simulink model "quadr_function"  (R2025b)
settings: Solver=VariableStepAuto  StartTime=0.0  StopTime=20  RelTol=1e-3
undefined symbols (not defined in the file or in its folder): K_att
libraries: mpclib x1
settings Model: Creator=abhay  LastModifiedBy=abhay

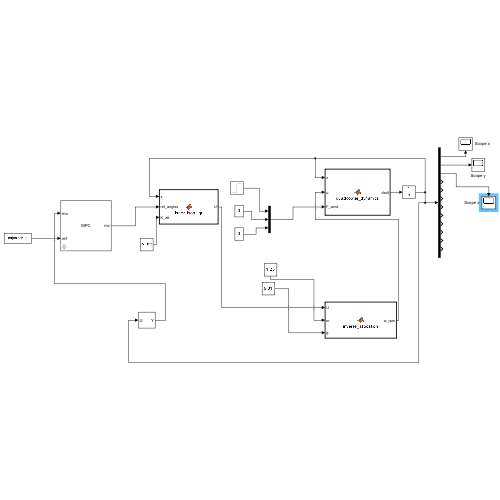
[thumbnail: Simulink's stored preview of the top-level diagram]
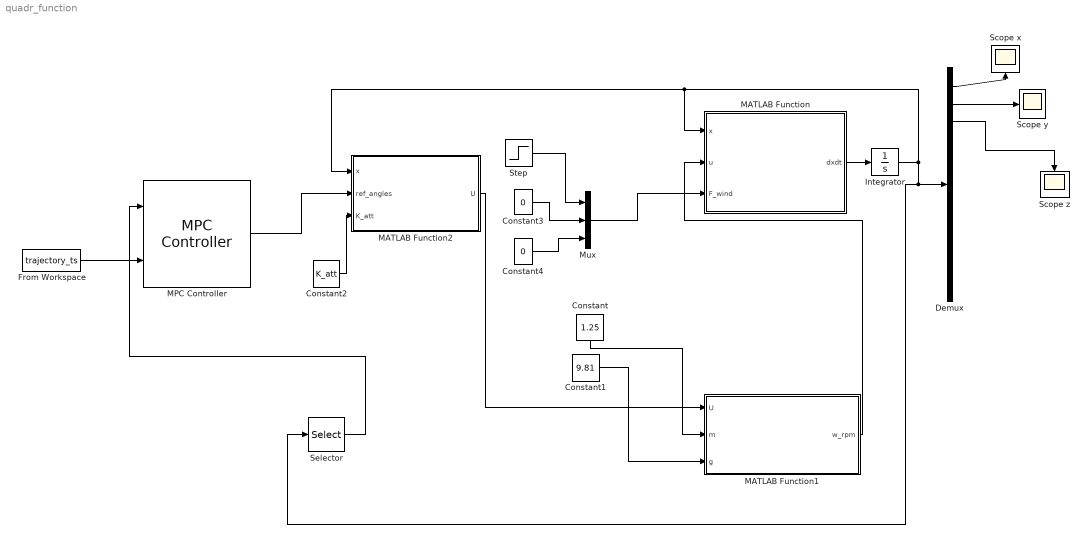
== system quadr_function ==
  Constant : Constant  Value=1.25
  Constant1 : Constant  Value=9.81
  Constant2 : Constant  Value=K_att  VectorParams1D=off
  Constant3 : Constant  Value=0
  Constant4 : Constant  Value=0
  Demux : Demux  Outputs=12
  From Workspace : FromWorkspace  VariableName=trajectory_ts
  Integrator : Integrator  InitialCondition=[2; 0; 10; 0; 1.0; 0.5; 0; 0; 0; 0; 0; 0]
  MATLAB Function : MATLAB Function  TreatAsAtomicUnit=on
  MATLAB Function1 : MATLAB Function  TreatAsAtomicUnit=on
  MATLAB Function2 : MATLAB Function  TreatAsAtomicUnit=on
  MPC Controller : mpclib/MPC Controller  SCDEnableBlockLinearizationSpecification=on  mpcobj=mpcobj  is_multiple=0  enable_value=0  return_u0=off  updateMPCinCallerWorkspace=on  md_inport=off  mv_inport=off  uref_inport=off  return_cost=off  return_mvseq=off  return_qpstatus=off  return_xseq=off  return_state=off  return_ovseq=off  state_inport=off  umin_inport=off  umax_inport=off  ymin_inport=off  ymax_inport=off  cc_inport=off  ywt_inport=off  uwt_inport=off  duwt_inport=off  rhoeps_inport=off  pm_inport=off  MaximumP=10  HorizonChoice=FixedHorizon  n_ts=0.05  n_p=20  n_mv=3  n_md=0  n_ud=0  n_mo=6  n_uo=0  BlockDataType=double  SampleTimeInherited=off  switch_inport=off
  Mux : Mux  Inputs=3
  Scope x : Scope
      settings: ActiveDisplayYMinimum=-2.7941018527251096  ActiveDisplayYMaximum=4.9347071430988949
  Scope y : Scope
      settings: ActiveDisplayYMinimum=-2.5407023374929745  ActiveDisplayYMaximum=2.8649607262454286
  Scope z : Scope
      settings: ActiveDisplayYMinimum=2.3361238691948745  ActiveDisplayYMaximum=21.3531300896177  DataLoggingVariableName=ScopeData2
  Selector : Selector  InputPortWidth=12  IndexOptions=Index vector (dialog)  Indices=[1 2 3 4 5 6]  OutputSizes=1
  Step : Step  Time=5  After=4  SampleTime=0
  wires:
  MATLAB Function/1(dxdt) -> Integrator/1
  Demux/1 -> Scope x/1
  Demux/2 -> Scope y/1
  Demux/3 -> Scope z/1
  MATLAB Function1/1(w_rpm) -> MATLAB Function/2(u)
  Constant/1 -> MATLAB Function1/2(m)
  Constant1/1 -> MATLAB Function1/3(g)
  MATLAB Function2/1(U) -> MATLAB Function1/1(U)
  Constant2/1 -> MATLAB Function2/3(K_att)
  MPC Controller/1 -> MATLAB Function2/2(ref_angles)
  From Workspace/1 -> MPC Controller/2
  Integrator/1 -> MATLAB Function2/1(x), MATLAB Function/1(x), Demux/1, Selector/1
  Selector/1 -> MPC Controller/1
  Step/1 -> Mux/1
  Constant3/1 -> Mux/2
  Constant4/1 -> Mux/3
  Mux/1 -> MATLAB Function/3(F_wind)

== matlab function quadr_function/MATLAB Function ==
  data: x input; u input; dxdt output; F_wind input
function dxdt = quadcopter_dynamics(x, u, F_wind)
    % x: State vector [12x1]
    % u: Control inputs [4x1] (Motor speeds in RPM)
    
    % --- 1. Physical Parameters (DJI F450) ---
    m = 1.250;              % Mass (kg)
    l = 0.235;              % Arm length (m)
    g = 9.81;               % Gravity (m/s^2)
    
    % Inertia Matrix (kg*m^2)
    Ixx = 0.0094;
    Iyy = 0.0100;
    Izz = 0.0187;
    
    % Aerodynamic Coefficients
    kf = 1.0155e-7;         % Thrust coefficient (N/RPM^2)
    km = 3.46e-8;           % Torque coefficient (N*m/RPM^2)

    % --- 2. Unpack State Vector ---
    % Position (Inertial Frame)
    pos = x(1:3);           % [x; y; z]
    % Velocity (Inertial Frame)
    vel = x(4:6);           % [xdot; ydot; zdot]
    % Euler Angles (Roll, Pitch, Yaw)
    phi = x(7);             
    theta = x(8);           
    psi = x(9);             
    % Angular Velocities (Body Frame)
    p = x(10);              
    q = x(11);              
    r = x(12);              

    % --- 3. Control Allocation (Motor Mixing) ---
    w1 = u(1); w2 = u(2); w3 = u(3); w4 = u(4);
    
    % Sum of squares of rotor speeds
    w_sq = [w1^2; w2^2; w3^2; w4^2];
    
    % U1: Total Thrust (Z-direction in Body Frame)
    U1 = kf * (w1^2 + w2^2 + w3^2 + w4^2);
    
    % U2, U3, U4: Roll, Pitch, Yaw Torques
    U2 = kf * l * (w4^2 + w1^2 - w2^2 - w3^2);
    U3 = kf * l * (w3^2 + w4^2 - w1^2 - w2^2);
    U4 = km * (w2^2 + w4^2 - w1^2 - w3^2);
    
    tau = [U2; U3; U4];     % Torque vector

    % --- 4. Translational Dynamics ---
    % Rotation Matrix (Body to Inertial) using Z-Y-X sequence
    R = [cos(psi)*cos(theta), cos(psi)*sin(theta)*sin(phi) - sin(psi)*cos(phi), cos(psi)*sin(theta)*cos(phi) + sin(psi)*sin(phi);
         sin(psi)*cos(theta), sin(psi)*sin(theta)*sin(phi) + cos(psi)*cos(phi), sin(psi)*sin(theta)*cos(phi) - cos(psi)*sin(phi);
         -sin(theta),         cos(theta)*sin(phi),                              cos(theta)*cos(phi)];
    
    % Gravity vector (Inertial Frame, Z is UP)
    F_gravity = [0; 0; -m*g];
    
    % Thrust vector (Body Frame, pushing UP)
    F_thrust_body = [0; 0; U1];
    
    % Acceleration (Inertial Frame)
    accel = (1/m) * (F_gravity + R * F_thrust_body + F_wind);

    % --- 5. Rotational Dynamics ---
    % Euler Angle Derivatives mapping matrix
    W = [1, sin(phi)*tan(theta), cos(phi)*tan(theta);
         0, cos(phi),           -sin(phi);
         0, sin(phi)/cos(theta), cos(phi)/cos(theta)];
    
    euler_rates = W * [p; q; r];
    
    % Angular Acceleration (Euler's Equation)
    % J * omega_dot = tau - cross(omega, J * omega)
    J = diag([Ixx, Iyy, Izz]);
    omega = [p; q; r];
    
    omega_dot = inv(J) * (tau - cross(omega, J * omega));

    % --- 6. Pack State Derivatives ---
    dxdt = zeros(12,1);
    dxdt(1:3)   = vel;              % Position derivatives (Velocity)
    dxdt(4:6)   = accel;            % Velocity derivatives (Acceleration)
    dxdt(7:9)   = euler_rates;      % Euler angle derivatives
    dxdt(10:12) = omega_dot;        % Angular velocity derivatives
end

== matlab function quadr_function/MATLAB Function2 ==
  data: x input; U output; ref_angles input; K_att input
function U = inner_loop_lqr(x, ref_angles, K_att)
    % x: Full 12x1 state vector from the plant
    % ref_angles: [theta_cmd; phi_cmd; delta_U1] from MPC
    
    % Extract current attitude states: [phi, theta, psi, p, q, r]
    x_att = x(7:12);
    
    % Extract commands from MPC
    theta_cmd = ref_angles(1);
    phi_cmd = ref_angles(2);
    delta_U1 = ref_angles(3);
    
    % Desired attitude vector (Assuming we want Yaw = 0, and rates = 0)
    x_att_ref = [phi_cmd; theta_cmd; 0; 0; 0; 0];
    
    % Calculate Error
    error = x_att - x_att_ref;
    
    % LQR Control Law: u = -K * error
    torques = -K_att * error;
    
    % Output [delta_U1; U2; U3; U4] to the Mixer
    U = [delta_U1; torques(1); torques(2); torques(3)];
end

== matlab function quadr_function/MATLAB Function1 ==
  data: U input; w_rpm output; m input; g input
function w_rpm = inverse_allocation(U, m, g)
    % U is a 4x1 vector: [delta_U1; U2; U3; U4]
    
    kf = 1.0155e-7;
    km = 3.46e-8;
    l = 0.235;
    
    % The MPC outputs deviation from hover thrust. We must add hover thrust back.
    U1_total = U(1) + (m * g); 
    U2 = U(2);
    U3 = U(3);
    U4 = U(4);
    
    % Allocation Matrix mapping W_squared to U
    M = [kf,      kf,      kf,      kf;
         kf*l,   -kf*l,   -kf*l,    kf*l;
        -kf*l,   -kf*l,    kf*l,    kf*l;
        -km,      km,     -km,      km];
        
    % Solve for Motor Speeds Squared
    W_sq = inv(M) * [U1_total; U2; U3; U4];
    
    % Prevent imaginary numbers if negative speeds are commanded
    W_sq(W_sq < 0) = 0; 
    
    % Convert back to RPM
    w_rpm = sqrt(W_sq);
end
